simulink model "Lazo_de_corrientes"  (R2023b)
settings: Solver=VariableStepAuto  StartTime=0.0  StopTime=10.0  RelTol=1e-3
undefined symbols (not defined in the file): R_0, R_d, R_q
settings Model: Creator=MSI  LastModifiedBy=MSI

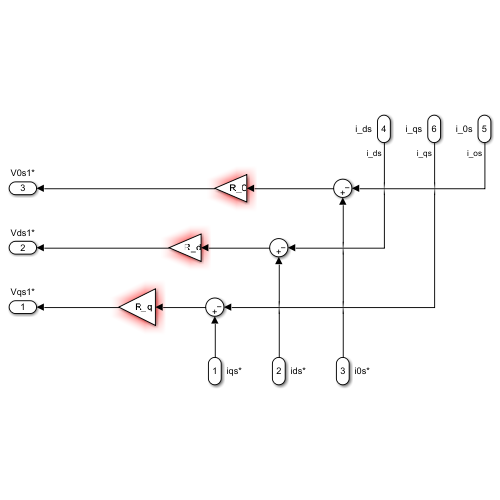
[thumbnail: Simulink's stored preview of the top-level diagram]
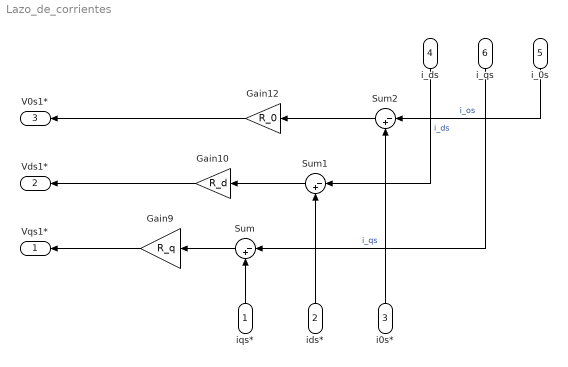
== system Lazo_de_corrientes ==
  iqs* : Inport
  ids* : Inport  Port=2
  i0s* : Inport  Port=3
  i_ds : Inport  Port=4
  i_0s : Inport  Port=5
  i_qs : Inport  Port=6
  Gain10 : Gain  Gain=R_d
  Gain12 : Gain  Gain=R_0
  Gain9 : Gain  Gain=R_q
  Sum : Sum  Inputs=|-+
  Sum1 : Sum  Inputs=|-+
  Sum2 : Sum  Inputs=|-+
  Vqs1* : Outport
  Vds1* : Outport  Port=2
  V0s1* : Outport  Port=3
  wires:
  Gain9/1 -> Vqs1*/1
  i_ds/1 -> Sum1/1  "i_ds"
  ids*/1 -> Sum1/2
  Sum/1 -> Gain9/1
  Sum2/1 -> Gain12/1
  Sum1/1 -> Gain10/1
  Gain10/1 -> Vds1*/1
  Gain12/1 -> V0s1*/1
  iqs*/1 -> Sum/2
  i_0s/1 -> Sum2/1  "i_os"
  i0s*/1 -> Sum2/2
  i_qs/1 -> Sum/1  "i_qs"
